simulink model "pmwtostm"  (R2024a)
settings: Solver=FixedStepAuto  StartTime=0.0  StopTime=0.1  FixedStep=1/400  RelTol=1e-3  EnableMultiTasking=on
model workspace (MAT data in the model file):
  MyHz = 8000
libraries: stm32f4xxblockslib x6, stm32h7xxblockslib x2, stm32blockslib x2
settings Model: STM32="{\"DigitalPortRead\":[{\"ID\":\"pmwtostm:93\"},{\"ID\":\"pmwtostm:115\"},{\"ID\":\"pmwtostm:116\"},{\"ID\":\"pmwtostm:117\"},{\"ID\":\"pmwtostm:118\"},{\"ID\":\"pmwtostm:119\"}],\"UdpSend\":{\"ID\":\"pmwtostm:96\"},\"UdpReceive\":{\"ID\":\"pmwtostm:133\"},\"PWMOutput\":[{\"ID\":\"pmwtostm:130\"},{\"ID\":\"pmwtostm:143\"}]}"  Creator=Konstantin  LastModifiedBy=Konstantin
settings OptimizationCC: EnhancedBackFolding=on  PassReuseOutputArgsAs=Individual arguments  ZeroExternalMemoryAtStartup=off  ZeroInternalMemoryAtStartup=off  MaxStackSize=64  OptimizeBlockOrder=speed  DifferentSizesBufferReuse=on  OptimizationCustomize=off  EfficientTunableParamExpr=on
settings DebuggingCC: ParameterTunabilityLossMsg=error
settings HardwareCC: ProdBitPerPointer=32  ProdBitPerSizeT=32  ProdBitPerPtrDiffT=32  ProdLargestAtomicInteger=Long  ProdLargestAtomicFloat=Double  ProdWordSize=32  ProdLongLongMode=on  ProdHWDeviceType=ARM Compatible->ARM Cortex-M
settings SFSimCC: MATLABDynamicMemAlloc=off
settings RTWCC: Description=Embedded Coder  SystemTargetFile=ert.tlc  HardwareBoard=STM32H7xx Based (Single-core)  TemplateMakefile=ert_default_tmf  Toolchain=GNU Tools for ARM Embedded Processors
settings CodeAppCC: ForceParamTrailComments=on  IgnoreCustomStorageClasses=off  OperatorAnnotations=on  SimulinkDataObjDesc=on  SFDataObjDesc=on  InsertBlockDesc=on
settings ERTTargetCC: TargetLangStandard=C99 (ISO)  CodeReplacementLibrary=ARM Cortex-M  ExtModeTransport=3  ExtModeStaticAlloc=on  ExtModeStaticAllocSize=2048  ExtModeMexFile=ext_xcp  ExtModeIntrfLevel=Level2 - Open

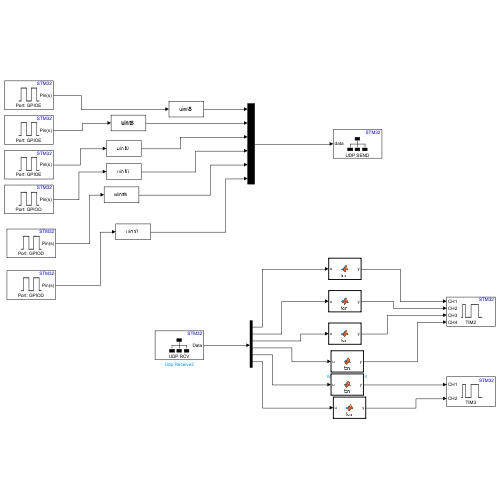
[thumbnail: Simulink's stored preview of the top-level diagram]
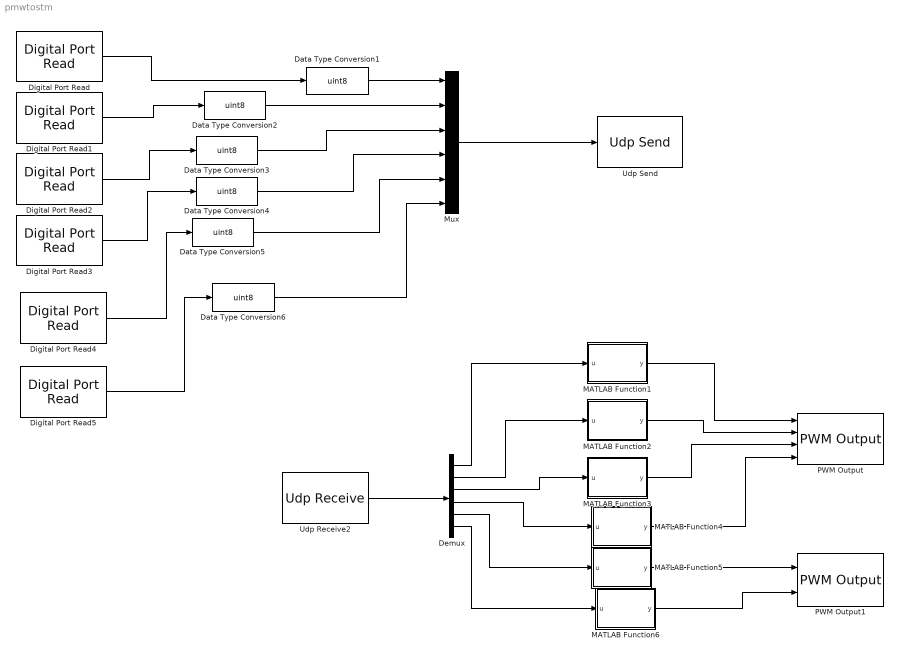
== system pmwtostm ==
  Data Type Conversion{1..6} (6 alike) : DataTypeConversion  OutDataTypeStr=uint8  SaturateOnIntegerOverflow=off  RndMeth=Floor
  Demux : Demux  Outputs=6
  Digital Port Read : stm32f4xxblockslib/Digital Port Read  PortName=GPIOE  PinNumber=[9]  ReadOperation=on  IOAsArray=on  SampleTime=1/400  EnableSimPort=off  hoistedMaskSrc=ECSoC/ECSimCodegen/Digital Port Read
      settings: LibrarySourceBlock=stm32h7xxblockslib/Digital Port Read
  Digital Port Read1 : stm32f4xxblockslib/Digital Port Read  PortName=GPIOE  PinNumber=[11]  ReadOperation=on  IOAsArray=on  SampleTime=1/400  EnableSimPort=off  hoistedMaskSrc=ECSoC/ECSimCodegen/Digital Port Read
      settings: LibrarySourceBlock=stm32h7xxblockslib/Digital Port Read
  Digital Port Read2 : stm32f4xxblockslib/Digital Port Read  PortName=GPIOE  PinNumber=[13]  ReadOperation=on  IOAsArray=on  SampleTime=1/400  EnableSimPort=off  hoistedMaskSrc=ECSoC/ECSimCodegen/Digital Port Read
      settings: LibrarySourceBlock=stm32h7xxblockslib/Digital Port Read
  Digital Port Read3 : stm32f4xxblockslib/Digital Port Read  PortName=GPIOD  PinNumber=[11]  ReadOperation=on  IOAsArray=on  SampleTime=1/400  EnableSimPort=off  hoistedMaskSrc=ECSoC/ECSimCodegen/Digital Port Read
      settings: LibrarySourceBlock=stm32h7xxblockslib/Digital Port Read
  Digital Port Read4 : stm32f4xxblockslib/Digital Port Read  PortName=GPIOD  PinNumber=[12]  ReadOperation=on  IOAsArray=on  SampleTime=1/400  EnableSimPort=off  hoistedMaskSrc=ECSoC/ECSimCodegen/Digital Port Read
      settings: LibrarySourceBlock=stm32h7xxblockslib/Digital Port Read
  Digital Port Read5 : stm32f4xxblockslib/Digital Port Read  PortName=GPIOD  PinNumber=[13]  ReadOperation=on  IOAsArray=on  SampleTime=1/400  EnableSimPort=off  hoistedMaskSrc=ECSoC/ECSimCodegen/Digital Port Read
      settings: LibrarySourceBlock=stm32h7xxblockslib/Digital Port Read
  MATLAB Function1 : MATLAB Function  TreatAsAtomicUnit=on
  MATLAB Function2 : MATLAB Function  TreatAsAtomicUnit=on
  MATLAB Function3 : MATLAB Function  TreatAsAtomicUnit=on
  MATLAB Function4 : MATLAB Function  TreatAsAtomicUnit=on
  MATLAB Function5 : MATLAB Function  TreatAsAtomicUnit=on
  MATLAB Function6 : MATLAB Function  TreatAsAtomicUnit=on
  Mux : Mux  Inputs=6
  PWM Output : stm32h7xxblockslib/PWM Output  TimerModule=TIM2  DutycycleUnits=Percentage  EnableChannel1=on  EnableChannel2=on  EnableChannel3=on  EnableChannel4=on  EnableChannel5=off  EnableChannel6=off  EnableCounterInput=off  EnableMainOutputInput=off  EnableFrequencyInput=off  SetRCAfterCE=off  OutputDirection=off  OutputMainOutputEnableStatus=off  SampleTime=0.1  EnableSimPort=off  EnableUpdateEvent=off  EnableCaptureCompare1Event=off  EnableCaptureCompare2Event=off  EnableCaptureCompare3Event=off  EnableCaptureCompare4Event=off  EnableTriggerEvent=off  EnableBreakEvent=off  EnableBreakEvent2=off  ProcessorFamily=STM32H7  hoistedMaskSrc=ECSoC/ECSimCodegen/PWM Output
  PWM Output1 : stm32h7xxblockslib/PWM Output  TimerModule=TIM3  DutycycleUnits=Percentage  EnableChannel1=on  EnableChannel2=on  EnableChannel3=off  EnableChannel4=off  EnableChannel5=off  EnableChannel6=off  EnableCounterInput=off  EnableMainOutputInput=off  EnableFrequencyInput=off  SetRCAfterCE=off  OutputDirection=off  OutputMainOutputEnableStatus=off  SampleTime=0.1  EnableSimPort=off  EnableUpdateEvent=off  EnableCaptureCompare1Event=off  EnableCaptureCompare2Event=off  EnableCaptureCompare3Event=off  EnableCaptureCompare4Event=off  EnableTriggerEvent=off  EnableBreakEvent=off  EnableBreakEvent2=off  ProcessorFamily=STM32H7  hoistedMaskSrc=ECSoC/ECSimCodegen/PWM Output
  Udp Receive2 : stm32blockslib/Udp Receive  Direction=Receive  RemoteIPAddress=192.168.1.2  LocalPort=25011  RemoteIPPort=25002  ByteOrder=LittleEndian  BlockingMode=off  BlockTimeout=0.1  DataType=double  DataLength=6  OutputStatus=off  SampleTime=-1
      settings: LibrarySourceBlock=stm32h7xxblockslib/Udp Receive
  Udp Send : stm32blockslib/Udp Send  Direction=Send  RemoteIPAddress=192.168.1.2  LocalPort=25010  RemoteIPPort=25002  ByteOrder=LittleEndian  BlockingMode=off  BlockTimeout=0.1  DataType=uint8  DataLength=1  OutputStatus=off
      settings: LibrarySourceBlock=stm32h7xxblockslib/Udp Send
  wires:
  Digital Port Read/1 -> Data Type Conversion1/1
  Mux/1 -> Udp Send/1
  Data Type Conversion1/1 -> Mux/1
  Data Type Conversion2/1 -> Mux/2
  Data Type Conversion3/1 -> Mux/3
  Data Type Conversion4/1 -> Mux/4
  Data Type Conversion5/1 -> Mux/5
  Data Type Conversion6/1 -> Mux/6
  Digital Port Read1/1 -> Data Type Conversion2/1
  Digital Port Read2/1 -> Data Type Conversion3/1
  Digital Port Read3/1 -> Data Type Conversion4/1
  Digital Port Read4/1 -> Data Type Conversion5/1
  Digital Port Read5/1 -> Data Type Conversion6/1
  MATLAB Function1/1(y) -> PWM Output/1
  Udp Receive2/1 -> Demux/1
  MATLAB Function2/1(y) -> PWM Output/2
  MATLAB Function3/1(y) -> PWM Output/3
  Demux/1 -> MATLAB Function1/1(u)
  Demux/2 -> MATLAB Function2/1(u)
  Demux/3 -> MATLAB Function3/1(u)
  Demux/4 -> MATLAB Function4/1(u)
  MATLAB Function4/1(y) -> PWM Output/4
  Demux/5 -> MATLAB Function5/1(u)
  MATLAB Function5/1(y) -> PWM Output1/1
  Demux/6 -> MATLAB Function6/1(u)
  MATLAB Function6/1(y) -> PWM Output1/2

== matlab function pmwtostm/MATLAB Function2 ==
  data: u input; y output
function y = fcn(u)

y = (u+2.5)/5*100;

== matlab function pmwtostm/MATLAB Function3 ==
  data: u input; y output
function y = fcn(u)

y = (u+2.5)/5*100;

== matlab function pmwtostm/MATLAB Function4 ==
  data: u input; y output
function y = fcn(u)

y = (u+40)/80*100;

== matlab function pmwtostm/MATLAB Function5 ==
  data: u input; y output
function y = fcn(u)

y = (u+40)/80*100;

== matlab function pmwtostm/MATLAB Function6 ==
  data: u input; y output
function y = fcn(u)

y = (u+40)/80*100;

== matlab function pmwtostm/MATLAB Function1 ==
  data: u input; y output
function y = fcn(u)

y = (u+2.5)/5*100;
